simulink model "x0toinc_EPOS4_R2020a"  (R2020a)
settings: Solver=ode4  StartTime=0.0  StopTime=inf  FixedStep=0.001  RelTol=1e-3
model workspace (MATLAB code in the model file):
  | x0toinc_EPOS4_ModelWorkspace;
values from neighbouring files (symbols this model uses):
  enc_pulse = 1000    [x0toinc_EPOS4_ModelWorkspace.m]
  Gear = 1    [x0toinc_EPOS4_ModelWorkspace.m]
  inc_center = 1000    [x0toinc_EPOS4_ModelWorkspace.m]
  Serial_mode = 2    [x0toinc_EPOS4_ModelWorkspace.m]
undefined symbols (not defined in the file or in its folder): LF, serial, Serial_Port, Standard_Devices
libraries: sldrtlib x3, instrumentlib x2, simulink_extras x1, simulink x1
settings Model: Creator=monami  LastModifiedBy=Monami
settings DataIOCC: SaveOutput=off  SignalLogging=off  DSMLogging=off  SaveTime=off  ReturnWorkspaceOutputs=off
settings RTWCC: Description=Simulink Desktop Real-Time  SystemTargetFile=sldrt.tlc  TemplateMakefile=sldrt.tmf  RTWCompilerOptimization=on
settings CodeAppCC: MaxIdLength=95
settings SimulinkDesktopRealTimeCC: TargetPreCompLibLocation=C:\Program Files\MATLAB\R2020b\toolbox\sldrt\lib\win64

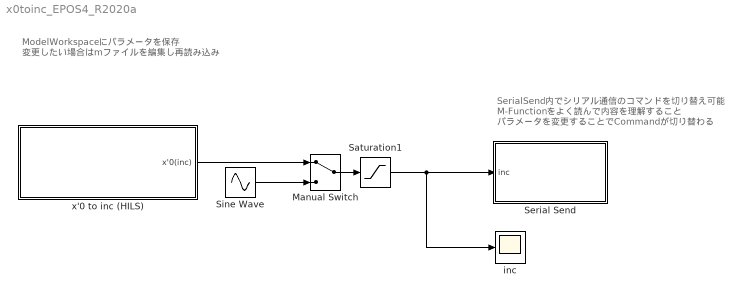
== system x0toinc_EPOS4_R2020a ==
  note: ModelWorkspaceにパラメータを保存
      | 変更したい場合はmファイルを編集し再読み込み
  note: SerialSend内でシリアル通信のコマンドを切り替え可能
      | M-Functionをよく読んで内容を理解すること
      | パラメータを変更することでCommandが切り替わる
  Manual Switch : ManualSwitch
  Saturation1 : Saturate  UpperLimit=47000  LowerLimit=0
  Serial Send : Subsystem
  Sine Wave : Sin  Amplitude=500  Bias=1000  SampleTime=0
  inc : Scope
  x'0 to inc (HILS) : Subsystem
  wires:
  Saturation1/1 -> Serial Send/1(inc), inc/1
  x'0 to inc (HILS)/1(x'0(inc)) -> Manual Switch/1
  Sine Wave/1 -> Manual Switch/2
  Manual Switch/1 -> Saturation1/1

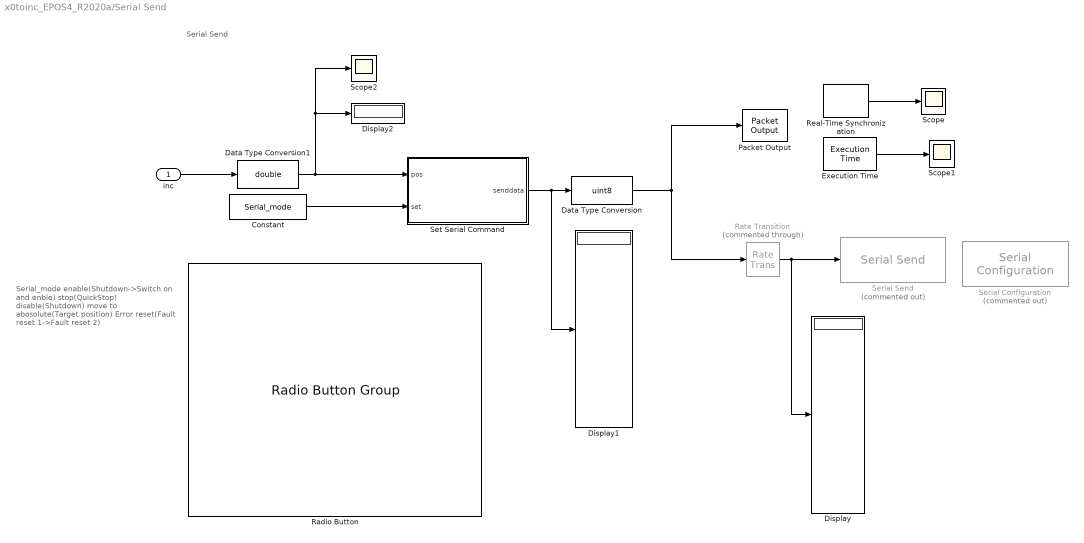
== system x0toinc_EPOS4_R2020a/Serial Send ==
  note: Serial_mode
      | enable(Shutdown->Switch on and enble)
      | stop(QuickStop)
      | disable(Shutdown)
      | move to abosolute(Target position)
      | Error reset(Fault reset 1->Fault reset 2)
  note: Serial Send
  inc : Inport
  Constant : Constant  Value=Serial_mode
  Data Type Conversion : DataTypeConversion  OutDataTypeStr=uint8
  Data Type Conversion1 : DataTypeConversion  OutDataTypeStr=double  RndMeth=Ceiling
  Display : Display
  Display1 : Display
  Display2 : Display
  Execution Time : sldrtlib/Target Profiling/Execution Time  ShowTaskTimes=off
      settings: SourceProductBaseCode=WT
  Packet Output : sldrtlib/Packet Output  SampleTime=0.002  MaxMissedTicks=10  ShowMissedTicks=off  YieldWhenWaiting=off  DrvName=Standard_Devices/Serial_Port  DrvAddress=4  DrvOptions=[115200 8 0 0 0 0 0 0]  PacketSize=14  DataTypes='14*uint8'  ShowReady=off  ShowError=off  PacketID=1  ByteOrder=1  InitialValue=[]  FinalValue=[]
      settings: AttributesFormatString=Serial Port [4]
  Radio Button : RadioButtonGroup  LabelPosition=Hide  SelectedLabel=Shutdown  ButtonGroupName=Serial_mode
      settings: Values={{'Traget Position', 'Quick Stop', 'Shutdown', 'Switch on and Enable', 'Fault reset 1', 'Fault reset 2'}, [0 1 2 3 4 5]}
  Rate Transition : RateTransition  Commented=through  OutPortSampleTime=0.004
  Real-Time Synchronization : sldrtlib/Real-Time Synchronization  SampleTime=0.001  MaxMissedTicks=10  ShowMissedTicks=on  YieldWhenWaiting=off
  Scope : Scope
  Scope1 : Scope
  Scope2 : Scope
  Serial Configuration : instrumentlib/Serial Configuration  Priority=-200000  Commented=on  ComPortMenu=COM4  ComPort=COM4  ObjConstructor=serial('COM4');  BaudRate=115200  DataBits=8  Parity=none  StopBits=1  FlowControl=none  Timeout=10  ByteOrder=LittleEndian
  Serial Send : instrumentlib/Serial Send  Commented=on  ComPortMenu=COM4  ComPort=COM4  ObjConstructor=serial('COM4');  Terminator=LF ('\n')  EnableBlockingMode=on
  Set Serial Command : MATLAB Function  TreatAsAtomicUnit=on
  wires:
  inc/1 -> Data Type Conversion1/1
  Data Type Conversion1/1 -> Set Serial Command/1(pos), Scope2/1, Display2/1
  Set Serial Command/1(senddata) -> Display1/1, Data Type Conversion/1
  Data Type Conversion/1 -> Rate Transition/1, Packet Output/1
  Rate Transition/1 -> Serial Send/1, Display/1
  Constant/1 -> Set Serial Command/2(set)
  Real-Time Synchronization/1 -> Scope/1
  Execution Time/1 -> Scope1/1

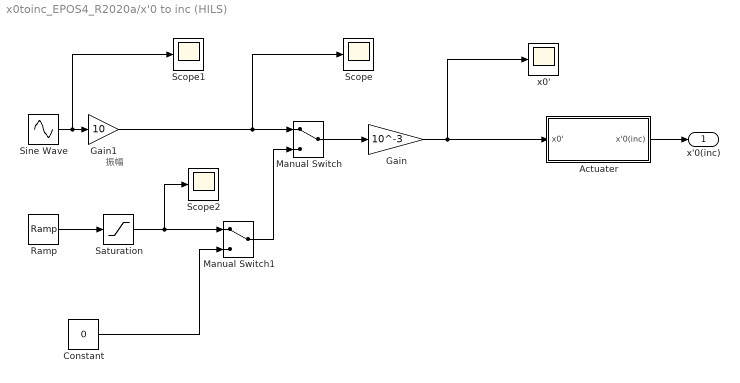
== system x0toinc_EPOS4_R2020a/x'0 to inc (HILS) ==
  note: 振幅
  Actuater : Subsystem
  Constant : Constant  Value=0
  Gain : Gain  Gain=10^-3
  Gain1 : Gain  Gain=10
  Manual Switch : ManualSwitch
  Manual Switch1 : ManualSwitch
  Ramp : simulink/Sources/Ramp  slope=200  start=10  InitialOutput=0
  Saturation : Saturate  UpperLimit=2000  LowerLimit=0
  Scope : Scope
  Scope1 : Scope
  Scope2 : Scope
  Sine Wave : Sin  Frequency=2*pi*1  SampleTime=0
  x0' : Scope
  x'0(inc) : Outport
  wires:
  Gain/1 -> x0'/1, Actuater/1(x0')
  Manual Switch/1 -> Gain/1
  Gain1/1 -> Scope/1, Manual Switch/1
  Sine Wave/1 -> Scope1/1, Gain1/1
  Saturation/1 -> Scope2/1, Manual Switch1/1
  Manual Switch1/1 -> Manual Switch/2
  Constant/1 -> Manual Switch1/2
  Ramp/1 -> Saturation/1
  Actuater/1(x'0(inc)) -> x'0(inc)/1

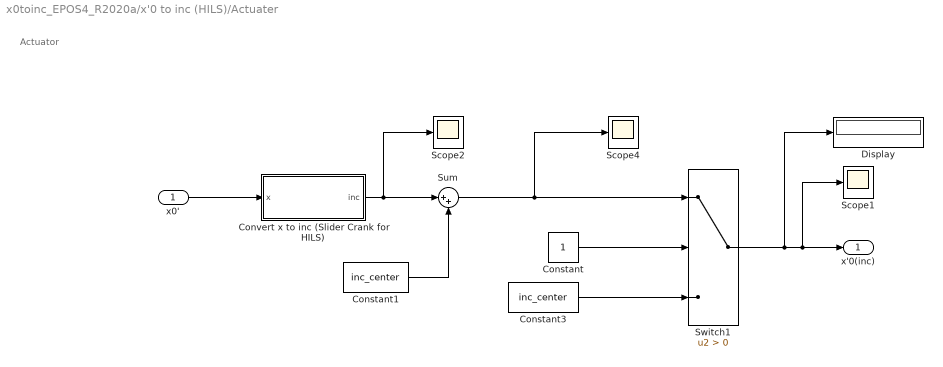
== system x0toinc_EPOS4_R2020a/x'0 to inc (HILS)/Actuater ==
  note: Actuator
  x0' : Inport
  Constant : Constant
  Constant1 : Constant  Value=inc_center
  Constant3 : Constant  Value=inc_center
  Convert x to inc (Slider Crank for HILS) : Subsystem
  Display : Display
  Scope1 : Scope
  Scope2 : Scope
  Scope4 : Scope
  Sum : Sum  Inputs=|++
  Switch1 : Switch  Criteria=u2 > Threshold
  x'0(inc) : Outport  VectorParamsAs1DForOutWhenUnconnected=off
  wires:
  Constant3/1 -> Switch1/3
  Constant/1 -> Switch1/2
  Switch1/1 -> Display/1, Scope1/1, x'0(inc)/1
  Sum/1 -> Scope4/1, Switch1/1
  x0'/1 -> Convert x to inc (Slider Crank for HILS)/1(x)
  Constant1/1 -> Sum/2
  Convert x to inc (Slider Crank for HILS)/1(inc) -> Scope2/1, Sum/1

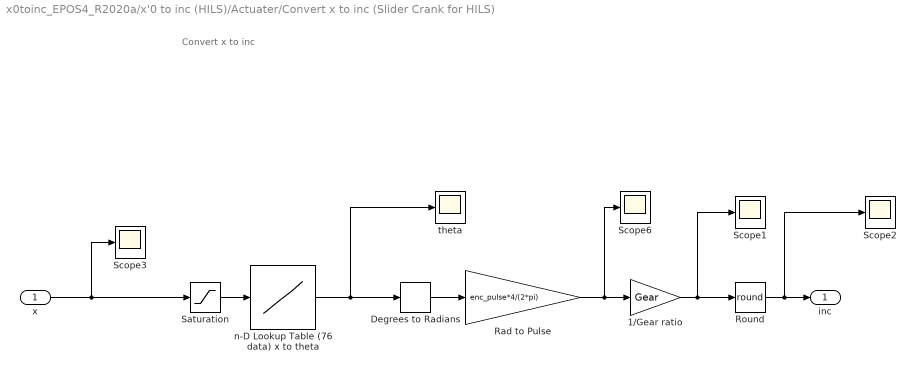
== system x0toinc_EPOS4_R2020a/x'0 to inc (HILS)/Actuater/Convert x to inc (Slider Crank for HILS) ==
  note: Convert x to inc
  x : Inport
  1/Gear ratio : Gain  Gain=Gear
  Degrees to Radians : simulink_extras/Transformations/Degrees to Radians
  Rad to Pulse : Gain  Gain=enc_pulse*4/(2*pi)
  Round : Rounding  Operator=round
  Saturation : Saturate  UpperLimit=0.03  LowerLimit=-0.03
  Scope{1..3,6} (4 alike) : Scope
  n-D Lookup Table (76 data) x to theta : Lookup_n-D  NumberOfTableDimensions=1  BreakpointsForDimension1=|  BreakpointsForDimension3=[5, 7]  Table=|  InterpMethod=Cubic spline  ExtrapMethod=Cubic spline  InternalRulePriority=Speed  RndMeth=Simplest  InputSameDT=on
      BreakpointsForDimension1=|
      | [-0.0306093330479605
      | -0.0298607961151376
      | -0.0291025282464357
      | -0.0283346628578736
      | -0.0275573426690830
      | -0.0267707198475020
      | -0.0259749561376706
      | -0.0251702229748870
      | -0.0243567015825286
      | -0.0235345830523965
      | -0.0227040684074941
      | -0.0218653686467141
      | -0.0210187047709721
      | -0.0201643077903933
      | -0.0193024187122293
      | -0.0184332885092591
      | -0.0175571780685010
      | -0.0166743581201432
      | -0.0157851091466777
      | -0.0148897212723015
      | -0.0139884941327283
      | -0.0130817367256312
      | -0.0121697672420139
      | -0.0112529128788804
      | -0.0103315096336475
      | -0.00940590208080894
      | -0.00847644313142852
      | -0.00754349377609770
      | -0.00660742281204917
      | -0.00566860655517083
      | -0.00472742853770840
      | -0.00378427919248757
      | -0.00283955552452070
      | -0.00189366077089287
      | -0.000947004049846267
      | 0
      | 0.000946931589344974
      | 0.00189336615585881
      | 0.00283887474883468
      | 0.00378302441988457
      | 0.00472537861873026
      | 0.00566549759315704
      | 0.00660293879220994
      | 0.00753725727173787
      | 0.00846800610141296
      | 0.00939473677238070
      | 0.0103169996047283
      | 0.0112343441539907
      | 0.0121463196159505
      | 0.0130524752290230
      | 0.0139523606735602
      | 0.0148455264674415
      | 0.0157315243573662
      | 0.0166099077052967
      | 0.0174802318695488
      | 0.0183420545800597
      | 0.0191949363074120
      | 0.0200384406252241
      | 0.0208721345655628
      | 0.0216955889670666
      | 0.0225083788155083
      | 0.0233100835765593
      | 0.0241002875205506
      | 0.0248785800390604
      | 0.0256445559531854
      | 0.0263978158133847
      | 0.0271379661908100
      | 0.0278646199600626
      | 0.0285773965733392
      | 0.0292759223259534
      | 0.0299598306132350
      | 0.0306287621788332
      | 0.0312823653544604
      | 0.0319202962911328
      | 0.0325422191819738
      | 0.0331478064766607]
      Table=|
      | [-15
      | -14
      | -13
      | -12
      | -11
      | -10
      | -9
      | -8
      | -7
      | -6
      | -5
      | -4
      | -3
      | -2
      | -1
      | 0
      | 1
      | 2
      | 3
      | 4
      | 5
      | 6
      | 7
      | 8
      | 9
      | 10
      | 11
      | 12
      | 13
      | 14
      | 15
      | 16
      | 17
      | 18
      | 19
      | 20
      | 21
      | 22
      | 23
      | 24
      | 25
      | 26
      | 27
      | 28
      | 29
      | 30
      | 31
      | 32
      | 33
      | 34
      | 35
      | 36
      | 37
      | 38
      | 39
      | 40
      | 41
      | 42
      | 43
      | 44
      | 45
      | 46
      | 47
      | 48
      | 49
      | 50
      | 51
      | 52
      | 53
      | 54
      | 55
      | 56
      | 57
      | 58
      | 59
      | 60]
  theta : Scope
  inc : Outport  VectorParamsAs1DForOutWhenUnconnected=off
  wires:
  1/Gear ratio/1 -> Scope1/1, Round/1
  Round/1 -> Scope2/1, inc/1
  Rad to Pulse/1 -> Scope6/1, 1/Gear ratio/1
  n-D Lookup Table (76 data) x to theta/1 -> theta/1, Degrees to Radians/1
  Saturation/1 -> n-D Lookup Table (76 data) x to theta/1
  Degrees to Radians/1 -> Rad to Pulse/1
  x/1 -> Scope3/1, Saturation/1

== matlab function x0toinc_EPOS4_R2020a/Serial Send/Set Serial Command ==
  data: pos input; senddata output; set input
function senddata = setSerialCommand(pos,set)
%Sets the state to switched on and enabled. Releases any Quickstop
%Build request frame

senddata = uint16(zeros(14,1));

switch set
    case 0
        senddata = func_sendTargetPosition(pos);
    case 1
        Controlword = '0002'; % Quick Stop
        senddata = setDeviceControlCommands(Controlword);
    case 2
        Controlword = '0006'; % Shutdown
        senddata = setDeviceControlCommands(Controlword);
    case 3
        Controlword = '000F'; % Switch on and enable
        senddata = setDeviceControlCommands(Controlword);
    case 4
        Controlword = '0000'; % Fault reset 1
        senddata = setDeviceControlCommands(Controlword);
    case 5
        Controlword = '0080'; % Fault reset 2
        senddata = setDeviceControlCommands(Controlword);
end
end

function senddata = setDeviceControlCommands(Controlword)
%Sets the state to switched on and enabled. Releases any Quickstop
%Build request frame

%SYNC: The first two bytes are used for frame synchronization.(EPOS4)
%   “DLE” (Data Link Escape) = 0x90
%   “STX” (Start of Text) = 0x02
DLE = uint16(0x90);
STX = uint16(0x02);
% DLE = uint16(myhex2dec('90'));
% STX = uint16(myhex2dec('02'));

%HEADER: The header consists of 2 bytes. The first field determines the type of data frame to be sent or received. The next field contains the length of the data fields.
%   "OpCode"(write) = 0x68
%   "Len" = 0x04
OpCode = uint16(0x68);
Len = uint16(0x04);
% OpCode = uint16(myhex2dec('68'));
% Len = uint16(myhex2dec('04'));


%% QuickStop: EPOS Node 1
%DATA: The data fields contain the parameters of the message. The low byte of the word is transmitted first.
%   NodeID = 0x01
%   Index of Object (Controlword): 0x6040
%   Subindex of Object = 0x00
%   device control command = 0x0002 0x0000

% DATA = uint16([myhex2dec('01') myhex2dec('40') myhex2dec('60') myhex2dec('00') myhex2dec(Controlword(3:4)) myhex2dec(Controlword(1:2)) myhex2dec('00') myhex2dec('00')]);
% DATAforCRC = uint16([myhex2dec('0468') myhex2dec('4001') myhex2dec('0060') myhex2dec(Controlword(1:4)) myhex2dec('0000')  myhex2dec('0000')]);
DATA = uint16([0x01 0x40 0x60 0x00 myhex2dec(Controlword(3:4)) myhex2dec(Controlword(1:2)) 0x00 0x00]);
DATAforCRC = uint16([0x0468 0x4001 0x0060 myhex2dec(Controlword(1:4)) 0x0000 0x0000]);
numberofWordsCRC = Len+2;
crc_hex = dec2hex(CRCcalc(DATAforCRC, numberofWordsCRC),4);
CRC = uint16([myhex2dec(crc_hex(3:4)) myhex2dec(crc_hex(1:2))]);

senddata=[DLE STX OpCode Len DATA CRC]';
end

function senddata = func_sendTargetPosition(pos)
%Sets the TargetPosition for Profile Position mode
%pos must be an integer.
% pos_hex = '';

if pos >= 0
    pos_hex = dec2hex(pos, 8);
else
    pos_hex = dec2hex(2^32+pos, 8);
end

%% Build write object request frame EPOS Node 1
%SYNC: The first two bytes are used for frame synchronization.(EPOS4)
%   “DLE” (Data Link Escape) = 0x90
%   “STX” (Start of Text) = 0x02
DLE = uint16(0x90);
STX = uint16(0x02);
% DLE = uint16(myhex2dec('90'));
% STX = uint16(myhex2dec('02'));

%HEADER: The header consists of 2 bytes. The first field determines the type of data frame to be sent or received. The next field contains the length of the data fields.
%   "OpCode"(write) = 0x68
%   "Len" = 0x04
OpCode = uint16(0x68);
Len = uint16(0x04);
% OpCode = uint16(myhex2dec('68'));
% Len = uint16(myhex2dec('04'));

%DATA: The data fields contain the parameters of the message. The low byte of the word is transmitted first.
%   NodeID = 0x01
%   Index of Object (Target Position): 0x607A
%   Subindex of Object = 0x00
%   Data byte to write[4]: pos_hex(1:4), pos_hex(5:8)

% DATA = uint16([myhex2dec('01') myhex2dec('7A') myhex2dec('60') myhex2dec('00') myhex2dec(pos_hex(7:8)) myhex2dec(pos_hex(5:6)) myhex2dec(pos_hex(3:4)) myhex2dec(pos_hex(1:2))]);
% DATAforCRC = uint16([myhex2dec('0468') myhex2dec('7A01') myhex2dec('0060') myhex2dec(pos_hex(5:8)) myhex2dec(pos_hex(1:4)) myhex2dec('0000')]);
DATA = uint16([0x01 0x7A 0x60 0x00 myhex2dec(pos_hex(7:8)) myhex2dec(pos_hex(5:6)) myhex2dec(pos_hex(3:4)) myhex2dec(pos_hex(1:2))]);
DATAforCRC = uint16([0x0468 0x7A01 0x0060 myhex2dec(pos_hex(5:8)) myhex2dec(pos_hex(1:4)) 0x0000]);
numberofWordsCRC = Len+2;
crc_hex = dec2hex(CRCcalc(DATAforCRC, numberofWordsCRC),4);
CRC = uint16([myhex2dec(crc_hex(3:4)) myhex2dec(crc_hex(1:2))]);

% senddata=[opCode Len_1 DATA CRC char('O')];
% senddata=[opCode Len_1 DATA CRC 79 10]';
senddata=[DLE STX OpCode Len DATA CRC]';
end

function d = myhex2dec(h)
%HEX2DEC Convert hexadecimal string to decimal integer.
%   this is the hex2dec function from Matlab with some checking disabled
%   for faster performance

if iscellstr(h), h = char(h); end
if isempty(h), d = []; return, end

% Work in upper case. - disabled since upper case anyways
%h = upper(h);

[m,n]=size(h);

% Right justify strings and form 2-D character array.
if ~isempty(find((h==' ' | h==0),1))
  h = strjust(h);

  % Replace any leading blanks and nulls by 0.
  h(cumsum(h ~= ' ' & h ~= 0,2) == 0) = '0';
else
  h = reshape(h,m,n);
end

% Check for out of range values - disabled
% if any(any(~((h>='0' & h<='9') | (h>='A'&h<='F'))))
%    error(message('MATLAB:hex2dec:IllegalHexadecimal'));
% end

sixteen = 16;
p = fliplr(cumprod([1 sixteen(ones(1,n-1))]));
p = p(ones(m,1),:);

d = h <= 64; % Numbers
h(d) = h(d) - 48;

d =  h > 64; % Letters
h(d) = h(d) - 55;

d = sum(h.*p,2);


end

function [ CRC ] = CRCcalc(DataArray, CRCnumberOfWords)
%Calculates the 16 bit CRC checksum according to communication guide for
%EPOS2
%Arguments are the DataArray that is being sent (opCode to Data) and the
%number of words

CRC = uint16(0);
for i=1:CRCnumberOfWords
    
    %shifter = uint16(myhex2dec('8000'));
    shifter = uint16(32768);
    c = DataArray(i);
    
    while(shifter)
        %carry = bitand(CRC, uint16(myhex2dec('8000')), 'uint16');
        carry = bitand(CRC, uint16(32768), 'uint16');
        CRC = bitshift(CRC,1,'uint16');
        if(bitand(c, shifter, 'uint16'))
            CRC = CRC +  1;
        end
        if(carry)
            %CRC = bitxor(CRC,uint16(myhex2dec('1021')),'uint16');
            CRC = bitxor(CRC,uint16(4129),'uint16');
        end
        shifter = bitshift(shifter,-1,'uint16');
    end
    
end


end
